simulink model "ScriptDemo"  (R2022b)
settings: configuration reference "TmVcThermal_Configuration_sub" (kept outside this file)
undefined symbols (not defined in the file or in its folder): aaaa, bbbb, cTmComprCtrl_D_u8HvacFlowTable_db, cTmComprCtrl_D_u8HvacFlowTable_sw, cTmComprCtrl_n_i16ChillCmpIMax, cTmComprCtrl_n_i16ChillCmpIMin, cTmComprCtrl_n_i16ChillCmpIMin666, cTmComprCtrl_n_i16ChillCmpPMax, cTmComprCtrl_n_i16ChillCmpPMin, cTmComprCtrl_n_i16CmpChillCoolRpmKiMax, cTmComprCtrl_n_i16CmpChillCoolRpmKiMin, cTmComprCtrl_n_i16CmpChillCoolRpmKpMax, cTmComprCtrl_n_i16CmpChillCoolRpmKpMin, cTmComprCtrl_n_i16CmpCoolRpmKiMax, cTmComprCtrl_n_i16CmpCoolRpmKiMin, cTmComprCtrl_n_i16CmpCoolRpmKpMax, cTmComprCtrl_n_i16CmpCoolRpmKpMin, cTmComprCtrl_n_i16SM4CmpHeatKiMax, cTmComprCtrl_n_i16SM4CmpHeatKiMin, cTmComprCtrl_n_i16SM4CmpHeatKpMax, cTmComprCtrl_n_i16SM4CmpHeatKpMin, cTmComprCtrl_n_i16SM5CmpHeatKiMax, cTmComprCtrl_n_i16SM5CmpHeatKiMin, cTmComprCtrl_n_i16SM5CmpHeatKpMax, cTmComprCtrl_n_i16SM5CmpHeatKpMin, cTmComprCtrl_n_i16SM6CmpHeatKiMax, cTmComprCtrl_n_i16SM6CmpHeatKiMin, cTmComprCtrl_n_i16SM6CmpHeatKpMax, cTmComprCtrl_n_i16SM6CmpHeatKpMin, cTmComprCtrl_n_u16CmpMaxSpdFanFltLimt, cTmComprCtrl_n_u16CmpMaxSpdLoSidePFltLimt, cTmComprCtrl_n_u16CmpMaxSpdSensorFltLimt, cTmComprCtrl_n_u16CompMinRpm, cTmComprCtrl_n_u16CompRpmIncThres, cTmComprCtrl_t_u16BattCooltFFPeriod, cTmComprCtrl_t_u16BattCooltPIPeriod, cTmComprCtrl_t_u16CmpCoolFFPeriod, cTmComprCtrl_t_u16CmpCoolPIPeriod, cTmComprCtrl_t_u16CoolCmpChillFFPeriod, cTmComprCtrl_t_u16CoolCmpChillPIPeriod, cTmComprCtrl_t_u16SM4CmpHeatFFPeriod, cTmComprCtrl_t_u16SM4CmpHeatPIPeriod, cTmComprCtrl_t_u16SM5CmpHeatFFPeriod, cTmComprCtrl_t_u16SM5CmpHeatPIPeriod, cTmComprCtrl_t_u16SM6CmpHeatFFPeriod, cTmComprCtrl_t_u16SM6CmpHeatPIPeriod, cTmComprCtrl_Te_EvapClearInteg, cTmComprCtrl_Te_i16HpReqTempSaturoffset, cTmComprCtrl_Te_i16SatLpReplaceDiff, cTmComprCtrl_Te_i16SM3BatDiffStartEvapDecOffset, cTmComprCtrl_Te_i16SM3EvapLo, cTmComprCtrl_Te_i16SM3TBatDiffEntEvapDecOffset, cTmComprCtrl_Te_i16SM3TBatDiffEntEvapDecOffsetQuit, cTmComprCtrl_Te_s32ErrCmpChillPIContinueCoolH, cTmComprCtrl_Te_s32ErrCmpChillPIContinueCoolL, cTmComprCtrl_Te_s32ErrCmpPIContinueChillH, cTmComprCtrl_Te_s32ErrCmpPIContinueChillL, cTmComprCtrl_Te_s32ErrCmpPIContinueCoolH, cTmComprCtrl_Te_s32ErrCmpPIContinueCoolL, cTmComprCtrl_Te_s32ErrCmpPIContinueHeatH ... (+398)
libraries: simulink x846, PCMULib x711, simulink_need_slupdate x4
(part 19 of 49)

== system ScriptDemo/Create/createBus/createBusGoto/After ==
  note: Before
  note: After
  TmComprCtrl : BusSelector  OutputSignals=Tasks.Task_100ms_TmSw.TmComprCtrl_100,TmDiag_Op.sTmDiag_D_u8BexvFltSt,TmDiag_Op.sTmDiag_D_u8CexvFltSt,TmDiag_Op.sTmDiag_D_u8EexvFltSt,TmDiag_Op.sTmDiag_D_u8FanFltSt,TmDiag_Op.sTmDiag_D_u8HiSidePFltSt,TmDiag_Op.sTmDiag_D_u8LoSidePFltSt,TmDiag_Op.sTmDiag_D_u8OutrCondOutTFltSt,TmDiag_Op.sTmDiag_D_u8Sov1FltSt,TmDiag_Op.sTmDiag_D_u8Sov2FltSt,TmDiag_Op.sTmDiag_D_u8Sov3FltSt,TmDiag_Op.sTmDiag_D_u8Sov4FltSt,TmDiag_Op.sTmDiag_D_u8Sov5FltSt,TmDiag_Op.sTmDiag_D_u8TeEvapFltSt,TmIn_Op.sTmIn_D_u8DCChrgSt,TmIn_Op.sTmIn_D_u8HeatPump,TmIn_Op.sTmIn_D_u8HvActvSts,TmIn_Op.sTmIn_I_s32ElacCmprHvActl,TmIn_Op.sTmIn_Pw_s32HvCoolgAllwd,TmIn_Op.sTmIn_Te_s32BattHv,TmSigProces_Op.sTmSigProces_Te_s32EvapFanReqRamp,TmIn_Op.sTmIn_Te_s32HvBattCooltT,TmIn_Op.sTmIn_Te_s32HvBattCooltTReq,TmIn_Op.sTmIn_U_s32ElacCmprHvActl,TmIn_Op.sTmIn_X_s32BexvPosSts,TmIn_Op.sTmIn_X_s32CexvPosSts,TmIn_Op.sTmIn_X_s32ClimtRcirc,TmIn_Op.sTmIn_X_s32EexvPosSts,TmIn_Op.sTmIn_X_s32HvacTFlpActlPosnFrtRowLe,TmIn_Op.sTmIn_X_s32HvacTFlpActlPosnFrtRowRi,TmIn_Op.sTmIn_n_s32ElacCmprActl,TmIn_Op.sTmIn_v_s32VehSpdLgt,TmRefriModeMgr_Op.sTmRefriModeMgr_D_u8HPCurMode,TmRefriModeMgr_Op.sTmRefriModeMgr_D_u8HpFmCmd,TmRefriModeMgr_Op.sTmRefriModeMgr_D_u8HpModeMainState,TmRefriVlvCtrl_Op.sTmRefriVlvCtrl_Z_u8BEXVInitState,TmRefriVlvCtrl_Op.sTmRefriVlvCtrl_Z_u8CEXVInitState,TmRefriVlvCtrl_Op.sTmRefriVlvCtrl_Z_u8EEXVInitState,TmSigProces_Op.sTmSigProces_D_u8BattThermReq,TmSigProces_Op.sTmSigProces_D_u8HvBattCoolgReq,TmSigProces_Op.sTmSigProces_D_u8PowerFault,TmSigProces_Op.sTmSigProces_Te_s32CompDischarge,TmSigProces_Op.sTmSigProces_Te_s32EvapFanFilter,TmSigProces_Op.sTmSigProces_Te_s32HeatrAirTReqRamp,TmSigProces_Op.sTmSigProces_Te_s32HvBattCooltTFilter,TmSigProces_Op.sTmSigProces_Te_s32HvBattCooltTOutFilter,TmSigProces_Op.sTmSigProces_Te_s32HvacHexAirTFilter,TmSigProces_Op.sTmSigProces_Te_s32TempInlet,TmSigProces_Op.sTmSigProces_Te_s32SatHp,TmSigProces_Op.sTmSigProces_Te_s32SatLp,TmSigProces_Op.sTmSigProces_md_u16BlwHeat,TmSigProces_Op.sTmSigProces_p_u16PHighSide,TmSigProces_Op.sTmSigProces_p_u16PLowSide,TmSovCtrl_Op.sTmSovCtrl_D_u8HpcSov1OnOffSts,TmSovCtrl_Op.sTmSovCtrl_D_u8HpcSov2OnOffSts,TmSovCtrl_Op.sTmSovCtrl_D_u8HpcSov3OnOffSts,TmSovCtrl_Op.sTmSovCtrl_D_u8HpcSov4OnOffSts,TmSovCtrl_Op.sTmSovCtrl_D_u8HpcSov5OnOffSts,TmHvchCtrl_Op.yTmHvchCtrl_B_HpcPtcEnad,TmIn_Op.yTmIn_B_ElAcEnable,TmRefriModeMgr_Op.yTmRefriModeMgr_B_CoolModeInCycle,TmSovCtrl_Op.yTmSovCtrl_B_HpmSov1ActvCmd,TmSovCtrl_Op.yTmSovCtrl_B_HpmSov2ActvCmd,TmSovCtrl_Op.yTmSovCtrl_B_HpmSov3ActvCmd,TmSovCtrl_Op.yTmSovCtrl_B_HpmSov4ActvCmd,TmSovCtrl_Op.yTmSovCtrl_B_HpmSov5ActvCmd,TmDiag_Op.sTmDiag_D_u8AccmFltSt,TmDiag_Op.sTmDiag_D_u8CmprPwrEna2FEnaState,TmDiag_Op.sTmDiag_D_u8CmprSpdEna2FEnaState,TmDiag_Op.sTmDiag_D_u8CmprStsEna2FEnaState,TmDiag_Op.sTmDiag_D_u8CmprStsEnaReq2F,TmDiag_Op.sTmDiag_D_u8HiSidePNHPFltSt,TmDiag_Op.sTmDiag_D_u8HvacHexAirTFltSt,TmDiag_Op.sTmDiag_D_u8InrCondOutTFltSt,TmDiag_Op.sTmDiag_D_u8RefrilackFltSt,TmDiag_Op.sTmDiag_Pw_s32CmprPwrEnaReq2F,TmDiag_Op.sTmDiag_n_s32CmprSpdReq2F,TmDiag_Op.sTmDiag_D_u8CmprDischrgTFltSt,TmSigProces_Op.sTmSigProces_Pw_i16ReqPwrForHeat,TmSigProces_Op.sTmSigProces_md_u16BlwCool,TmSigProces_Op.sTmSigProces_D_u8CarChrgMode,TmIn_Op.sTmIn_D_u8ElecDriveline,TmRefriModeMgr_Op.sTmRefriModeMgr_D_u8CabinCoolReq,TmRefriModeMgr_Op.sTmRefriModeMgr_D_u8CabinHeatReq,TmRefriModeMgr_Op.sTmRefriModeMgr_D_u8HpModeCmd,TmSigProces_Op.sTmSigProces_Te_s32TAmb,TmRefriModeMgr_Op.sTmRefriModeMgr_D_u8ModeSwitchType,TmRefriModeMgr_Op.yTmRefriModeMgr_B_CoolOCRMode,TmDiag_Op.sTmDiag_D_u8BattPmpFltSt,TmDiag_Op.sTmDiag_D_u8HvBattCooltTFltSt,TmDiag_Op.sTmDiag_D_u8HvBattCooltTOutFltSt,TmIn_Op.sTmIn_D_u8OnBdChrgrHndlSts,TmSigProces_Op.sTmSigProces_Pw_i16ReqPwrForCool,TmRefriModeMgr_Op.yTmRefriModeMgr_B_HeatModeInCycle
  TmComprCtrl1 : BusSelector  OutputSignals=Tasks.Task_100ms_TmSw.TmComprCtrl_100,TmDiag_Op.sTmDiag_D_u8BexvFltSt,TmDiag_Op.sTmDiag_D_u8CexvFltSt,TmDiag_Op.sTmDiag_D_u8EexvFltSt,TmDiag_Op.sTmDiag_D_u8FanFltSt,TmDiag_Op.sTmDiag_D_u8HiSidePFltSt,TmDiag_Op.sTmDiag_D_u8LoSidePFltSt,TmDiag_Op.sTmDiag_D_u8OutrCondOutTFltSt,TmDiag_Op.sTmDiag_D_u8Sov1FltSt,TmDiag_Op.sTmDiag_D_u8Sov2FltSt,TmDiag_Op.sTmDiag_D_u8Sov3FltSt,TmDiag_Op.sTmDiag_D_u8Sov4FltSt,TmDiag_Op.sTmDiag_D_u8Sov5FltSt,TmDiag_Op.sTmDiag_D_u8TeEvapFltSt,TmIn_Op.sTmIn_D_u8DCChrgSt,TmIn_Op.sTmIn_D_u8HeatPump,TmIn_Op.sTmIn_D_u8HvActvSts,TmIn_Op.sTmIn_I_s32ElacCmprHvActl,TmIn_Op.sTmIn_Pw_s32HvCoolgAllwd,TmIn_Op.sTmIn_Te_s32BattHv,TmSigProces_Op.sTmSigProces_Te_s32EvapFanReqRamp,TmIn_Op.sTmIn_Te_s32HvBattCooltT,TmIn_Op.sTmIn_Te_s32HvBattCooltTReq,TmIn_Op.sTmIn_U_s32ElacCmprHvActl,TmIn_Op.sTmIn_X_s32BexvPosSts,TmIn_Op.sTmIn_X_s32CexvPosSts,TmIn_Op.sTmIn_X_s32ClimtRcirc,TmIn_Op.sTmIn_X_s32EexvPosSts,TmIn_Op.sTmIn_X_s32HvacTFlpActlPosnFrtRowLe,TmIn_Op.sTmIn_X_s32HvacTFlpActlPosnFrtRowRi,TmIn_Op.sTmIn_n_s32ElacCmprActl,TmIn_Op.sTmIn_v_s32VehSpdLgt,TmRefriModeMgr_Op.sTmRefriModeMgr_D_u8HPCurMode,TmRefriModeMgr_Op.sTmRefriModeMgr_D_u8HpFmCmd,TmRefriModeMgr_Op.sTmRefriModeMgr_D_u8HpModeMainState,TmRefriVlvCtrl_Op.sTmRefriVlvCtrl_Z_u8BEXVInitState,TmRefriVlvCtrl_Op.sTmRefriVlvCtrl_Z_u8CEXVInitState,TmRefriVlvCtrl_Op.sTmRefriVlvCtrl_Z_u8EEXVInitState,TmSigProces_Op.sTmSigProces_D_u8BattThermReq,TmSigProces_Op.sTmSigProces_D_u8HvBattCoolgReq,TmSigProces_Op.sTmSigProces_D_u8PowerFault,TmSigProces_Op.sTmSigProces_Te_s32CompDischarge,TmSigProces_Op.sTmSigProces_Te_s32EvapFanFilter,TmSigProces_Op.sTmSigProces_Te_s32HeatrAirTReqRamp,TmSigProces_Op.sTmSigProces_Te_s32HvBattCooltTFilter,TmSigProces_Op.sTmSigProces_Te_s32HvBattCooltTOutFilter,TmSigProces_Op.sTmSigProces_Te_s32HvacHexAirTFilter,TmSigProces_Op.sTmSigProces_Te_s32TempInlet,TmSigProces_Op.sTmSigProces_Te_s32SatHp,TmSigProces_Op.sTmSigProces_Te_s32SatLp,TmSigProces_Op.sTmSigProces_md_u16BlwHeat,TmSigProces_Op.sTmSigProces_p_u16PHighSide,TmSigProces_Op.sTmSigProces_p_u16PLowSide,TmSovCtrl_Op.sTmSovCtrl_D_u8HpcSov1OnOffSts,TmSovCtrl_Op.sTmSovCtrl_D_u8HpcSov2OnOffSts,TmSovCtrl_Op.sTmSovCtrl_D_u8HpcSov3OnOffSts,TmSovCtrl_Op.sTmSovCtrl_D_u8HpcSov4OnOffSts,TmSovCtrl_Op.sTmSovCtrl_D_u8HpcSov5OnOffSts,TmHvchCtrl_Op.yTmHvchCtrl_B_HpcPtcEnad,TmIn_Op.yTmIn_B_ElAcEnable,TmRefriModeMgr_Op.yTmRefriModeMgr_B_CoolModeInCycle,TmSovCtrl_Op.yTmSovCtrl_B_HpmSov1ActvCmd,TmSovCtrl_Op.yTmSovCtrl_B_HpmSov2ActvCmd,TmSovCtrl_Op.yTmSovCtrl_B_HpmSov3ActvCmd,TmSovCtrl_Op.yTmSovCtrl_B_HpmSov4ActvCmd,TmSovCtrl_Op.yTmSovCtrl_B_HpmSov5ActvCmd,TmDiag_Op.sTmDiag_D_u8AccmFltSt,TmDiag_Op.sTmDiag_D_u8CmprPwrEna2FEnaState,TmDiag_Op.sTmDiag_D_u8CmprSpdEna2FEnaState,TmDiag_Op.sTmDiag_D_u8CmprStsEna2FEnaState,TmDiag_Op.sTmDiag_D_u8CmprStsEnaReq2F,TmDiag_Op.sTmDiag_D_u8HiSidePNHPFltSt,TmDiag_Op.sTmDiag_D_u8HvacHexAirTFltSt,TmDiag_Op.sTmDiag_D_u8InrCondOutTFltSt,TmDiag_Op.sTmDiag_D_u8RefrilackFltSt,TmDiag_Op.sTmDiag_Pw_s32CmprPwrEnaReq2F,TmDiag_Op.sTmDiag_n_s32CmprSpdReq2F,TmDiag_Op.sTmDiag_D_u8CmprDischrgTFltSt,TmSigProces_Op.sTmSigProces_Pw_i16ReqPwrForHeat,TmSigProces_Op.sTmSigProces_md_u16BlwCool,TmSigProces_Op.sTmSigProces_D_u8CarChrgMode,TmIn_Op.sTmIn_D_u8ElecDriveline,TmRefriModeMgr_Op.sTmRefriModeMgr_D_u8CabinCoolReq,TmRefriModeMgr_Op.sTmRefriModeMgr_D_u8CabinHeatReq,TmRefriModeMgr_Op.sTmRefriModeMgr_D_u8HpModeCmd,TmSigProces_Op.sTmSigProces_Te_s32TAmb,TmRefriModeMgr_Op.sTmRefriModeMgr_D_u8ModeSwitchType,TmRefriModeMgr_Op.yTmRefriModeMgr_B_CoolOCRMode,TmDiag_Op.sTmDiag_D_u8BattPmpFltSt,TmDiag_Op.sTmDiag_D_u8HvBattCooltTFltSt,TmDiag_Op.sTmDiag_D_u8HvBattCooltTOutFltSt,TmIn_Op.sTmIn_D_u8OnBdChrgrHndlSts,TmSigProces_Op.sTmSigProces_Pw_i16ReqPwrForCool,TmRefriModeMgr_Op.yTmRefriModeMgr_B_HeatModeInCycle
  wires:
  TmComprCtrl1/1 -> [TmComprCtrl_100]  "<TmComprCtrl_100>"
  TmComprCtrl1/2 -> [sTmDiag_D_u8BexvFltSt]  "<sTmDiag_D_u8BexvFltSt>"
  TmComprCtrl1/3 -> [sTmDiag_D_u8CexvFltSt]  "<sTmDiag_D_u8CexvFltSt>"
  TmComprCtrl1/4 -> [sTmDiag_D_u8EexvFltSt]  "<sTmDiag_D_u8EexvFltSt>"
  TmComprCtrl1/5 -> [sTmDiag_D_u8FanFltSt]  "<sTmDiag_D_u8FanFltSt>"
  TmComprCtrl1/6 -> [sTmDiag_D_u8HiSidePFltSt]  "<sTmDiag_D_u8HiSidePFltSt>"
  TmComprCtrl1/7 -> [sTmDiag_D_u8LoSidePFltSt]  "<sTmDiag_D_u8LoSidePFltSt>"
  TmComprCtrl1/8 -> [sTmDiag_D_u8OutrCondOutTFltSt]  "<sTmDiag_D_u8OutrCondOutTFltSt>"
  TmComprCtrl1/9 -> [sTmDiag_D_u8Sov1FltSt]  "<sTmDiag_D_u8Sov1FltSt>"
  TmComprCtrl1/10 -> [sTmDiag_D_u8Sov2FltSt]  "<sTmDiag_D_u8Sov2FltSt>"
  TmComprCtrl1/11 -> [sTmDiag_D_u8Sov3FltSt]  "<sTmDiag_D_u8Sov3FltSt>"
  TmComprCtrl1/12 -> [sTmDiag_D_u8Sov4FltSt]  "<sTmDiag_D_u8Sov4FltSt>"
  TmComprCtrl1/13 -> [sTmDiag_D_u8Sov5FltSt]  "<sTmDiag_D_u8Sov5FltSt>"
  TmComprCtrl1/14 -> [sTmDiag_D_u8TeEvapFltSt]  "<sTmDiag_D_u8TeEvapFltSt>"
  TmComprCtrl1/15 -> [sTmIn_D_u8DCChrgSt]  "<sTmIn_D_u8DCChrgSt>"
  TmComprCtrl1/16 -> [sTmIn_D_u8HeatPump]  "<sTmIn_D_u8HeatPump>"
  TmComprCtrl1/17 -> [sTmIn_D_u8HvActvSts]  "<sTmIn_D_u8HvActvSts>"
  TmComprCtrl1/18 -> [sTmIn_I_s32ElacCmprHvActl]  "<sTmIn_I_s32ElacCmprHvActl>"
  TmComprCtrl1/19 -> [sTmIn_Pw_s32HvCoolgAllwd]  "<sTmIn_Pw_s32HvCoolgAllwd>"
  TmComprCtrl1/20 -> [sTmIn_Te_s32BattHv]  "<sTmIn_Te_s32BattHv>"
  TmComprCtrl1/21 -> [sTmSigProces_Te_s32EvapFanReqRamp]  "<sTmSigProces_Te_s32EvapFanReqRamp>"
  TmComprCtrl1/22 -> [sTmIn_Te_s32HvBattCooltT]  "<sTmIn_Te_s32HvBattCooltT>"
  TmComprCtrl1/23 -> [sTmIn_Te_s32HvBattCooltTReq]  "<sTmIn_Te_s32HvBattCooltTReq>"
  TmComprCtrl1/24 -> [sTmIn_U_s32ElacCmprHvActl]  "<sTmIn_U_s32ElacCmprHvActl>"
  TmComprCtrl1/25 -> [sTmIn_X_s32BexvPosSts]  "<sTmIn_X_s32BexvPosSts>"
  TmComprCtrl1/26 -> [sTmIn_X_s32CexvPosSts]  "<sTmIn_X_s32CexvPosSts>"
  TmComprCtrl1/27 -> [sTmIn_X_s32ClimtRcirc]  "<sTmIn_X_s32ClimtRcirc>"
  TmComprCtrl1/28 -> [sTmIn_X_s32EexvPosSts]  "<sTmIn_X_s32EexvPosSts>"
  TmComprCtrl1/29 -> [sTmIn_X_s32HvacTFlpActlPosnFrtRowLe]  "<sTmIn_X_s32HvacTFlpActlPosnFrtRowLe>"
  TmComprCtrl1/30 -> [sTmIn_X_s32HvacTFlpActlPosnFrtRowRi]  "<sTmIn_X_s32HvacTFlpActlPosnFrtRowRi>"
  TmComprCtrl1/31 -> [sTmIn_n_s32ElacCmprActl]  "<sTmIn_n_s32ElacCmprActl>"
  TmComprCtrl1/32 -> [sTmIn_v_s32VehSpdLgt]  "<sTmIn_v_s32VehSpdLgt>"
  TmComprCtrl1/33 -> [sTmRefriModeMgr_D_u8HPCurMode]  "<sTmRefriModeMgr_D_u8HPCurMode>"
  TmComprCtrl1/34 -> [sTmRefriModeMgr_D_u8HpFmCmd]  "<sTmRefriModeMgr_D_u8HpFmCmd>"
  TmComprCtrl1/35 -> [sTmRefriModeMgr_D_u8HpModeMainState]  "<sTmRefriModeMgr_D_u8HpModeMainState>"
  TmComprCtrl1/36 -> [sTmRefriVlvCtrl_Z_u8BEXVInitState]  "<sTmRefriVlvCtrl_Z_u8BEXVInitState>"
  TmComprCtrl1/37 -> [sTmRefriVlvCtrl_Z_u8CEXVInitState]  "<sTmRefriVlvCtrl_Z_u8CEXVInitState>"
  TmComprCtrl1/38 -> [sTmRefriVlvCtrl_Z_u8EEXVInitState]  "<sTmRefriVlvCtrl_Z_u8EEXVInitState>"
  TmComprCtrl1/39 -> [sTmSigProces_D_u8BattThermReq]  "<sTmSigProces_D_u8BattThermReq>"
  TmComprCtrl1/40 -> [sTmSigProces_D_u8HvBattCoolgReq]  "<sTmSigProces_D_u8HvBattCoolgReq>"
  TmComprCtrl1/41 -> [sTmSigProces_D_u8PowerFault]  "<sTmSigProces_D_u8PowerFault>"
  TmComprCtrl1/42 -> [sTmSigProces_Te_s32CompDischarge]  "<sTmSigProces_Te_s32CompDischarge>"
  TmComprCtrl1/43 -> [sTmSigProces_Te_s32EvapFanFilter]  "<sTmSigProces_Te_s32EvapFanFilter>"
  TmComprCtrl1/44 -> [sTmSigProces_Te_s32HeatrAirTReqRamp]  "<sTmSigProces_Te_s32HeatrAirTReqRamp>"
  TmComprCtrl1/45 -> [sTmSigProces_Te_s32HvBattCooltTFilter]  "<sTmSigProces_Te_s32HvBattCooltTFilter>"
  TmComprCtrl1/46 -> [sTmSigProces_Te_s32HvBattCooltTOutFilter]  "<sTmSigProces_Te_s32HvBattCooltTOutFilter>"
  TmComprCtrl1/47 -> [sTmSigProces_Te_s32HvacHexAirTFilter]  "<sTmSigProces_Te_s32HvacHexAirTFilter>"
  TmComprCtrl1/48 -> [sTmSigProces_Te_s32TempInlet]  "<sTmSigProces_Te_s32TempInlet>"
  TmComprCtrl1/49 -> [sTmSigProces_Te_s32SatHp]  "<sTmSigProces_Te_s32SatHp>"
  TmComprCtrl1/50 -> [sTmSigProces_Te_s32SatLp]  "<sTmSigProces_Te_s32SatLp>"
  TmComprCtrl1/51 -> [sTmSigProces_md_u16BlwHeat]  "<sTmSigProces_md_u16BlwHeat>"
  TmComprCtrl1/52 -> [sTmSigProces_p_u16PHighSide]  "<sTmSigProces_p_u16PHighSide>"
  TmComprCtrl1/53 -> [sTmSigProces_p_u16PLowSide]  "<sTmSigProces_p_u16PLowSide>"
  TmComprCtrl1/54 -> [sTmSovCtrl_D_u8HpcSov1OnOffSts]  "<sTmSovCtrl_D_u8HpcSov1OnOffSts>"
  TmComprCtrl1/55 -> [sTmSovCtrl_D_u8HpcSov2OnOffSts]  "<sTmSovCtrl_D_u8HpcSov2OnOffSts>"
  TmComprCtrl1/56 -> [sTmSovCtrl_D_u8HpcSov3OnOffSts]  "<sTmSovCtrl_D_u8HpcSov3OnOffSts>"
  TmComprCtrl1/57 -> [sTmSovCtrl_D_u8HpcSov4OnOffSts]  "<sTmSovCtrl_D_u8HpcSov4OnOffSts>"
  TmComprCtrl1/58 -> [sTmSovCtrl_D_u8HpcSov5OnOffSts]  "<sTmSovCtrl_D_u8HpcSov5OnOffSts>"
  TmComprCtrl1/59 -> [yTmHvchCtrl_B_HpcPtcEnad]  "<yTmHvchCtrl_B_HpcPtcEnad>"
  TmComprCtrl1/60 -> [yTmIn_B_ElAcEnable]  "<yTmIn_B_ElAcEnable>"
  TmComprCtrl1/61 -> [yTmRefriModeMgr_B_CoolModeInCycle]  "<yTmRefriModeMgr_B_CoolModeInCycle>"
  TmComprCtrl1/62 -> [yTmSovCtrl_B_HpmSov1ActvCmd]  "<yTmSovCtrl_B_HpmSov1ActvCmd>"
  TmComprCtrl1/63 -> [yTmSovCtrl_B_HpmSov2ActvCmd]  "<yTmSovCtrl_B_HpmSov2ActvCmd>"
  TmComprCtrl1/64 -> [yTmSovCtrl_B_HpmSov3ActvCmd]  "<yTmSovCtrl_B_HpmSov3ActvCmd>"
  TmComprCtrl1/65 -> [yTmSovCtrl_B_HpmSov4ActvCmd]  "<yTmSovCtrl_B_HpmSov4ActvCmd>"
  TmComprCtrl1/66 -> [yTmSovCtrl_B_HpmSov5ActvCmd]  "<yTmSovCtrl_B_HpmSov5ActvCmd>"
  TmComprCtrl1/67 -> [sTmDiag_D_u8AccmFltSt]  "<sTmDiag_D_u8AccmFltSt>"
  TmComprCtrl1/68 -> [sTmDiag_D_u8CmprPwrEna2FEnaState]  "<sTmDiag_D_u8CmprPwrEna2FEnaState>"
  TmComprCtrl1/69 -> [sTmDiag_D_u8CmprSpdEna2FEnaState]  "<sTmDiag_D_u8CmprSpdEna2FEnaState>"
  TmComprCtrl1/70 -> [sTmDiag_D_u8CmprStsEna2FEnaState]  "<sTmDiag_D_u8CmprStsEna2FEnaState>"
  TmComprCtrl1/71 -> [sTmDiag_D_u8CmprStsEnaReq2F]  "<sTmDiag_D_u8CmprStsEnaReq2F>"
  TmComprCtrl1/72 -> [sTmDiag_D_u8HiSidePNHPFltSt]  "<sTmDiag_D_u8HiSidePNHPFltSt>"
  TmComprCtrl1/73 -> [sTmDiag_D_u8HvacHexAirTFltSt]  "<sTmDiag_D_u8HvacHexAirTFltSt>"
  TmComprCtrl1/74 -> [sTmDiag_D_u8InrCondOutTFltSt]  "<sTmDiag_D_u8InrCondOutTFltSt>"
  TmComprCtrl1/75 -> [sTmDiag_D_u8RefrilackFltSt]  "<sTmDiag_D_u8RefrilackFltSt>"
  TmComprCtrl1/76 -> [sTmDiag_Pw_s32CmprPwrEnaReq2F]  "<sTmDiag_Pw_s32CmprPwrEnaReq2F>"
  TmComprCtrl1/77 -> [sTmDiag_n_s32CmprSpdReq2F]  "<sTmDiag_n_s32CmprSpdReq2F>"
  TmComprCtrl1/78 -> [sTmDiag_D_u8CmprDischrgTFltSt]  "<sTmDiag_D_u8CmprDischrgTFltSt>"
  TmComprCtrl1/79 -> [sTmSigProces_Pw_i16ReqPwrForHeat]  "<sTmSigProces_Pw_i16ReqPwrForHeat>"
  TmComprCtrl1/80 -> [sTmSigProces_md_u16BlwCool]  "<sTmSigProces_md_u16BlwCool>"
  TmComprCtrl1/81 -> [sTmSigProces_D_u8CarChrgMode]  "<sTmSigProces_D_u8CarChrgMode>"
  TmComprCtrl1/82 -> [sTmIn_D_u8ElecDriveline]  "<sTmIn_D_u8ElecDriveline>"
  TmComprCtrl1/83 -> [sTmRefriModeMgr_D_u8CabinCoolReq]  "<sTmRefriModeMgr_D_u8CabinCoolReq>"
  TmComprCtrl1/84 -> [sTmRefriModeMgr_D_u8CabinHeatReq]  "<sTmRefriModeMgr_D_u8CabinHeatReq>"
  TmComprCtrl1/85 -> [sTmRefriModeMgr_D_u8HpModeCmd]  "<sTmRefriModeMgr_D_u8HpModeCmd>"
  TmComprCtrl1/86 -> [sTmSigProces_Te_s32TAmb]  "<sTmSigProces_Te_s32TAmb>"
  TmComprCtrl1/87 -> [sTmRefriModeMgr_D_u8ModeSwitchType]  "<sTmRefriModeMgr_D_u8ModeSwitchType>"
  TmComprCtrl1/88 -> [yTmRefriModeMgr_B_CoolOCRMode]  "<yTmRefriModeMgr_B_CoolOCRMode>"
  TmComprCtrl1/89 -> [sTmDiag_D_u8BattPmpFltSt]  "<sTmDiag_D_u8BattPmpFltSt>"
  TmComprCtrl1/90 -> [sTmDiag_D_u8HvBattCooltTFltSt]  "<sTmDiag_D_u8HvBattCooltTFltSt>"
  TmComprCtrl1/91 -> [sTmDiag_D_u8HvBattCooltTOutFltSt]  "<sTmDiag_D_u8HvBattCooltTOutFltSt>"
  TmComprCtrl1/92 -> [sTmIn_D_u8OnBdChrgrHndlSts]  "<sTmIn_D_u8OnBdChrgrHndlSts>"
  TmComprCtrl1/93 -> [sTmSigProces_Pw_i16ReqPwrForCool]  "<sTmSigProces_Pw_i16ReqPwrForCool>"
  TmComprCtrl1/94 -> [yTmRefriModeMgr_B_HeatModeInCycle]  "<yTmRefriModeMgr_B_HeatModeInCycle>"

== system ScriptDemo/Create/createBus/createBusGoto/Before ==
  TmComprCtrl : BusSelector  OutputSignals=Tasks.Task_100ms_TmSw.TmComprCtrl_100,TmDiag_Op.sTmDiag_D_u8BexvFltSt,TmDiag_Op.sTmDiag_D_u8CexvFltSt,TmDiag_Op.sTmDiag_D_u8EexvFltSt,TmDiag_Op.sTmDiag_D_u8FanFltSt,TmDiag_Op.sTmDiag_D_u8HiSidePFltSt,TmDiag_Op.sTmDiag_D_u8LoSidePFltSt,TmDiag_Op.sTmDiag_D_u8OutrCondOutTFltSt,TmDiag_Op.sTmDiag_D_u8Sov1FltSt,TmDiag_Op.sTmDiag_D_u8Sov2FltSt,TmDiag_Op.sTmDiag_D_u8Sov3FltSt,TmDiag_Op.sTmDiag_D_u8Sov4FltSt,TmDiag_Op.sTmDiag_D_u8Sov5FltSt,TmDiag_Op.sTmDiag_D_u8TeEvapFltSt,TmIn_Op.sTmIn_D_u8DCChrgSt,TmIn_Op.sTmIn_D_u8HeatPump,TmIn_Op.sTmIn_D_u8HvActvSts,TmIn_Op.sTmIn_I_s32ElacCmprHvActl,TmIn_Op.sTmIn_Pw_s32HvCoolgAllwd,TmIn_Op.sTmIn_Te_s32BattHv,TmSigProces_Op.sTmSigProces_Te_s32EvapFanReqRamp,TmIn_Op.sTmIn_Te_s32HvBattCooltT,TmIn_Op.sTmIn_Te_s32HvBattCooltTReq,TmIn_Op.sTmIn_U_s32ElacCmprHvActl,TmIn_Op.sTmIn_X_s32BexvPosSts,TmIn_Op.sTmIn_X_s32CexvPosSts,TmIn_Op.sTmIn_X_s32ClimtRcirc,TmIn_Op.sTmIn_X_s32EexvPosSts,TmIn_Op.sTmIn_X_s32HvacTFlpActlPosnFrtRowLe,TmIn_Op.sTmIn_X_s32HvacTFlpActlPosnFrtRowRi,TmIn_Op.sTmIn_n_s32ElacCmprActl,TmIn_Op.sTmIn_v_s32VehSpdLgt,TmRefriModeMgr_Op.sTmRefriModeMgr_D_u8HPCurMode,TmRefriModeMgr_Op.sTmRefriModeMgr_D_u8HpFmCmd,TmRefriModeMgr_Op.sTmRefriModeMgr_D_u8HpModeMainState,TmRefriVlvCtrl_Op.sTmRefriVlvCtrl_Z_u8BEXVInitState,TmRefriVlvCtrl_Op.sTmRefriVlvCtrl_Z_u8CEXVInitState,TmRefriVlvCtrl_Op.sTmRefriVlvCtrl_Z_u8EEXVInitState,TmSigProces_Op.sTmSigProces_D_u8BattThermReq,TmSigProces_Op.sTmSigProces_D_u8HvBattCoolgReq,TmSigProces_Op.sTmSigProces_D_u8PowerFault,TmSigProces_Op.sTmSigProces_Te_s32CompDischarge,TmSigProces_Op.sTmSigProces_Te_s32EvapFanFilter,TmSigProces_Op.sTmSigProces_Te_s32HeatrAirTReqRamp,TmSigProces_Op.sTmSigProces_Te_s32HvBattCooltTFilter,TmSigProces_Op.sTmSigProces_Te_s32HvBattCooltTOutFilter,TmSigProces_Op.sTmSigProces_Te_s32HvacHexAirTFilter,TmSigProces_Op.sTmSigProces_Te_s32TempInlet,TmSigProces_Op.sTmSigProces_Te_s32SatHp,TmSigProces_Op.sTmSigProces_Te_s32SatLp,TmSigProces_Op.sTmSigProces_md_u16BlwHeat,TmSigProces_Op.sTmSigProces_p_u16PHighSide,TmSigProces_Op.sTmSigProces_p_u16PLowSide,TmSovCtrl_Op.sTmSovCtrl_D_u8HpcSov1OnOffSts,TmSovCtrl_Op.sTmSovCtrl_D_u8HpcSov2OnOffSts,TmSovCtrl_Op.sTmSovCtrl_D_u8HpcSov3OnOffSts,TmSovCtrl_Op.sTmSovCtrl_D_u8HpcSov4OnOffSts,TmSovCtrl_Op.sTmSovCtrl_D_u8HpcSov5OnOffSts,TmHvchCtrl_Op.yTmHvchCtrl_B_HpcPtcEnad,TmIn_Op.yTmIn_B_ElAcEnable,TmRefriModeMgr_Op.yTmRefriModeMgr_B_CoolModeInCycle,TmSovCtrl_Op.yTmSovCtrl_B_HpmSov1ActvCmd,TmSovCtrl_Op.yTmSovCtrl_B_HpmSov2ActvCmd,TmSovCtrl_Op.yTmSovCtrl_B_HpmSov3ActvCmd,TmSovCtrl_Op.yTmSovCtrl_B_HpmSov4ActvCmd,TmSovCtrl_Op.yTmSovCtrl_B_HpmSov5ActvCmd,TmDiag_Op.sTmDiag_D_u8AccmFltSt,TmDiag_Op.sTmDiag_D_u8CmprPwrEna2FEnaState,TmDiag_Op.sTmDiag_D_u8CmprSpdEna2FEnaState,TmDiag_Op.sTmDiag_D_u8CmprStsEna2FEnaState,TmDiag_Op.sTmDiag_D_u8CmprStsEnaReq2F,TmDiag_Op.sTmDiag_D_u8HiSidePNHPFltSt,TmDiag_Op.sTmDiag_D_u8HvacHexAirTFltSt,TmDiag_Op.sTmDiag_D_u8InrCondOutTFltSt,TmDiag_Op.sTmDiag_D_u8RefrilackFltSt,TmDiag_Op.sTmDiag_Pw_s32CmprPwrEnaReq2F,TmDiag_Op.sTmDiag_n_s32CmprSpdReq2F,TmDiag_Op.sTmDiag_D_u8CmprDischrgTFltSt,TmSigProces_Op.sTmSigProces_Pw_i16ReqPwrForHeat,TmSigProces_Op.sTmSigProces_md_u16BlwCool,TmSigProces_Op.sTmSigProces_D_u8CarChrgMode,TmIn_Op.sTmIn_D_u8ElecDriveline,TmRefriModeMgr_Op.sTmRefriModeMgr_D_u8CabinCoolReq,TmRefriModeMgr_Op.sTmRefriModeMgr_D_u8CabinHeatReq,TmRefriModeMgr_Op.sTmRefriModeMgr_D_u8HpModeCmd,TmSigProces_Op.sTmSigProces_Te_s32TAmb,TmRefriModeMgr_Op.sTmRefriModeMgr_D_u8ModeSwitchType,TmRefriModeMgr_Op.yTmRefriModeMgr_B_CoolOCRMode,TmDiag_Op.sTmDiag_D_u8BattPmpFltSt,TmDiag_Op.sTmDiag_D_u8HvBattCooltTFltSt,TmDiag_Op.sTmDiag_D_u8HvBattCooltTOutFltSt,TmIn_Op.sTmIn_D_u8OnBdChrgrHndlSts,TmSigProces_Op.sTmSigProces_Pw_i16ReqPwrForCool,TmRefriModeMgr_Op.yTmRefriModeMgr_B_HeatModeInCycle

== system ScriptDemo/Create/createBus/createBusPort/After ==
  note: Before
  note: After
  TmComprCtrl : BusSelector  OutputSignals=TmSigProces_Op.sTmSigProces_Te_s32TempInlet,TmSigProces_Op.sTmSigProces_Te_s32SatHp,TmSigProces_Op.sTmSigProces_Te_s32SatLp,TmSigProces_Op.sTmSigProces_md_u16BlwHeat,TmSigProces_Op.sTmSigProces_p_u16PHighSide,TmSigProces_Op.sTmSigProces_p_u16PLowSide,TmSovCtrl_Op.sTmSovCtrl_D_u8HpcSov1OnOffSts,TmSovCtrl_Op.sTmSovCtrl_D_u8HpcSov2OnOffSts,TmSovCtrl_Op.sTmSovCtrl_D_u8HpcSov3OnOffSts,TmSovCtrl_Op.sTmSovCtrl_D_u8HpcSov4OnOffSts,TmSovCtrl_Op.sTmSovCtrl_D_u8HpcSov5OnOffSts,TmHvchCtrl_Op.yTmHvchCtrl_B_HpcPtcEnad,TmIn_Op.yTmIn_B_ElAcEnable,TmRefriModeMgr_Op.yTmRefriModeMgr_B_CoolModeInCycle,TmSovCtrl_Op.yTmSovCtrl_B_HpmSov1ActvCmd,TmSovCtrl_Op.yTmSovCtrl_B_HpmSov2ActvCmd,TmSovCtrl_Op.yTmSovCtrl_B_HpmSov3ActvCmd,TmSovCtrl_Op.yTmSovCtrl_B_HpmSov4ActvCmd,TmSovCtrl_Op.yTmSovCtrl_B_HpmSov5ActvCmd,TmDiag_Op.sTmDiag_D_u8AccmFltSt,TmDiag_Op.sTmDiag_D_u8CmprPwrEna2FEnaState,TmDiag_Op.sTmDiag_D_u8CmprSpdEna2FEnaState,TmDiag_Op.sTmDiag_D_u8CmprStsEna2FEnaState,TmDiag_Op.sTmDiag_D_u8CmprStsEnaReq2F,TmDiag_Op.sTmDiag_D_u8HiSidePNHPFltSt,TmDiag_Op.sTmDiag_D_u8HvacHexAirTFltSt,TmDiag_Op.sTmDiag_D_u8InrCondOutTFltSt,TmDiag_Op.sTmDiag_D_u8RefrilackFltSt,TmDiag_Op.sTmDiag_Pw_s32CmprPwrEnaReq2F,TmDiag_Op.sTmDiag_n_s32CmprSpdReq2F,TmDiag_Op.sTmDiag_D_u8CmprDischrgTFltSt,TmSigProces_Op.sTmSigProces_Pw_i16ReqPwrForHeat,TmSigProces_Op.sTmSigProces_md_u16BlwCool,TmSigProces_Op.sTmSigProces_D_u8CarChrgMode,TmIn_Op.sTmIn_D_u8ElecDriveline,TmRefriModeMgr_Op.sTmRefriModeMgr_D_u8CabinCoolReq,TmRefriModeMgr_Op.sTmRefriModeMgr_D_u8CabinHeatReq,TmRefriModeMgr_Op.sTmRefriModeMgr_D_u8HpModeCmd,TmSigProces_Op.sTmSigProces_Te_s32TAmb,TmRefriModeMgr_Op.sTmRefriModeMgr_D_u8ModeSwitchType,TmRefriModeMgr_Op.yTmRefriModeMgr_B_CoolOCRMode,TmDiag_Op.sTmDiag_D_u8BattPmpFltSt,TmDiag_Op.sTmDiag_D_u8HvBattCooltTFltSt,TmDiag_Op.sTmDiag_D_u8HvBattCooltTOutFltSt,TmIn_Op.sTmIn_D_u8OnBdChrgrHndlSts,TmSigProces_Op.sTmSigProces_Pw_i16ReqPwrForCool,TmRefriModeMgr_Op.yTmRefriModeMgr_B_HeatModeInCycle
  TmComprCtrl1 : BusSelector  OutputSignals=TmSigProces_Op.sTmSigProces_Te_s32TempInlet,TmSigProces_Op.sTmSigProces_Te_s32SatHp,TmSigProces_Op.sTmSigProces_Te_s32SatLp,TmSigProces_Op.sTmSigProces_md_u16BlwHeat,TmSigProces_Op.sTmSigProces_p_u16PHighSide,TmSigProces_Op.sTmSigProces_p_u16PLowSide,TmSovCtrl_Op.sTmSovCtrl_D_u8HpcSov1OnOffSts,TmSovCtrl_Op.sTmSovCtrl_D_u8HpcSov2OnOffSts,TmSovCtrl_Op.sTmSovCtrl_D_u8HpcSov3OnOffSts,TmSovCtrl_Op.sTmSovCtrl_D_u8HpcSov4OnOffSts,TmSovCtrl_Op.sTmSovCtrl_D_u8HpcSov5OnOffSts,TmHvchCtrl_Op.yTmHvchCtrl_B_HpcPtcEnad,TmIn_Op.yTmIn_B_ElAcEnable,TmRefriModeMgr_Op.yTmRefriModeMgr_B_CoolModeInCycle,TmSovCtrl_Op.yTmSovCtrl_B_HpmSov1ActvCmd,TmSovCtrl_Op.yTmSovCtrl_B_HpmSov2ActvCmd,TmSovCtrl_Op.yTmSovCtrl_B_HpmSov3ActvCmd,TmSovCtrl_Op.yTmSovCtrl_B_HpmSov4ActvCmd,TmSovCtrl_Op.yTmSovCtrl_B_HpmSov5ActvCmd,TmDiag_Op.sTmDiag_D_u8AccmFltSt,TmDiag_Op.sTmDiag_D_u8CmprPwrEna2FEnaState,TmDiag_Op.sTmDiag_D_u8CmprSpdEna2FEnaState,TmDiag_Op.sTmDiag_D_u8CmprStsEna2FEnaState,TmDiag_Op.sTmDiag_D_u8CmprStsEnaReq2F,TmDiag_Op.sTmDiag_D_u8HiSidePNHPFltSt,TmDiag_Op.sTmDiag_D_u8HvacHexAirTFltSt,TmDiag_Op.sTmDiag_D_u8InrCondOutTFltSt,TmDiag_Op.sTmDiag_D_u8RefrilackFltSt,TmDiag_Op.sTmDiag_Pw_s32CmprPwrEnaReq2F,TmDiag_Op.sTmDiag_n_s32CmprSpdReq2F,TmDiag_Op.sTmDiag_D_u8CmprDischrgTFltSt,TmSigProces_Op.sTmSigProces_Pw_i16ReqPwrForHeat,TmSigProces_Op.sTmSigProces_md_u16BlwCool,TmSigProces_Op.sTmSigProces_D_u8CarChrgMode,TmIn_Op.sTmIn_D_u8ElecDriveline,TmRefriModeMgr_Op.sTmRefriModeMgr_D_u8CabinCoolReq,TmRefriModeMgr_Op.sTmRefriModeMgr_D_u8CabinHeatReq,TmRefriModeMgr_Op.sTmRefriModeMgr_D_u8HpModeCmd,TmSigProces_Op.sTmSigProces_Te_s32TAmb,TmRefriModeMgr_Op.sTmRefriModeMgr_D_u8ModeSwitchType,TmRefriModeMgr_Op.yTmRefriModeMgr_B_CoolOCRMode,TmDiag_Op.sTmDiag_D_u8BattPmpFltSt,TmDiag_Op.sTmDiag_D_u8HvBattCooltTFltSt,TmDiag_Op.sTmDiag_D_u8HvBattCooltTOutFltSt,TmIn_Op.sTmIn_D_u8OnBdChrgrHndlSts,TmSigProces_Op.sTmSigProces_Pw_i16ReqPwrForCool,TmRefriModeMgr_Op.yTmRefriModeMgr_B_HeatModeInCycle
  sTmSigProces_Te_s32SatHp : Outport
  sTmSigProces_Te_s32SatLp : Outport  Port=2
  sTmSigProces_md_u16BlwHeat : Outport  Port=3
  sTmSigProces_p_u16PHighSide : Outport  Port=4
  sTmSigProces_p_u16PLowSide : Outport  Port=5
  sTmSovCtrl_D_u8HpcSov1OnOffSts : Outport  Port=6
  sTmSovCtrl_D_u8HpcSov2OnOffSts : Outport  Port=7
  sTmSovCtrl_D_u8HpcSov3OnOffSts : Outport  Port=8
  sTmSovCtrl_D_u8HpcSov4OnOffSts : Outport  Port=9
  sTmSovCtrl_D_u8HpcSov5OnOffSts : Outport  Port=10
  yTmHvchCtrl_B_HpcPtcEnad : Outport  Port=11
  yTmIn_B_ElAcEnable : Outport  Port=12
  yTmSovCtrl_B_HpmSov1ActvCmd : Outport  Port=13
  yTmSovCtrl_B_HpmSov2ActvCmd : Outport  Port=14
  yTmSovCtrl_B_HpmSov3ActvCmd : Outport  Port=15
  yTmSovCtrl_B_HpmSov4ActvCmd : Outport  Port=16
  yTmSovCtrl_B_HpmSov5ActvCmd : Outport  Port=17
  sTmDiag_D_u8AccmFltSt : Outport  Port=18
  sTmDiag_D_u8CmprPwrEna2FEnaState : Outport  Port=19
  sTmDiag_D_u8CmprSpdEna2FEnaState : Outport  Port=20
  sTmDiag_D_u8CmprStsEna2FEnaState : Outport  Port=21
  sTmDiag_D_u8CmprStsEnaReq2F : Outport  Port=22
  sTmDiag_D_u8HiSidePNHPFltSt : Outport  Port=23
  sTmDiag_D_u8HvacHexAirTFltSt : Outport  Port=24
  sTmDiag_D_u8InrCondOutTFltSt : Outport  Port=25
  sTmDiag_D_u8RefrilackFltSt : Outport  Port=26
  sTmDiag_Pw_s32CmprPwrEnaReq2F : Outport  Port=27
  sTmDiag_n_s32CmprSpdReq2F : Outport  Port=28
  sTmDiag_D_u8CmprDischrgTFltSt : Outport  Port=29
  sTmSigProces_Pw_i16ReqPwrForHeat : Outport  Port=30
  sTmSigProces_md_u16BlwCool : Outport  Port=31
  sTmIn_D_u8ElecDriveline : Outport  Port=32
  sTmRefriModeMgr_D_u8CabinCoolReq : Outport  Port=33
  sTmRefriModeMgr_D_u8CabinHeatReq : Outport  Port=34
  sTmRefriModeMgr_D_u8ModeSwitchType : Outport  Port=35
  yTmRefriModeMgr_B_CoolOCRMode : Outport  Port=36
  sTmDiag_D_u8BattPmpFltSt : Outport  Port=37
  sTmDiag_D_u8HvBattCooltTFltSt : Outport  Port=38
  sTmDiag_D_u8HvBattCooltTOutFltSt : Outport  Port=39
  sTmIn_D_u8OnBdChrgrHndlSts : Outport  Port=40
  sTmSigProces_Pw_i16ReqPwrForCool : Outport  Port=41
  yTmRefriModeMgr_B_HeatModeInCycle : Outport  Port=42
  wires:
  TmComprCtrl1/1 -> ?  "<sTmSigProces_Te_s32TempInlet>"
  TmComprCtrl1/2 -> sTmSigProces_Te_s32SatHp/1  "<sTmSigProces_Te_s32SatHp>"
  TmComprCtrl1/3 -> sTmSigProces_Te_s32SatLp/1  "<sTmSigProces_Te_s32SatLp>"
  TmComprCtrl1/4 -> sTmSigProces_md_u16BlwHeat/1  "<sTmSigProces_md_u16BlwHeat>"
  TmComprCtrl1/5 -> sTmSigProces_p_u16PHighSide/1  "<sTmSigProces_p_u16PHighSide>"
  TmComprCtrl1/6 -> sTmSigProces_p_u16PLowSide/1  "<sTmSigProces_p_u16PLowSide>"
  TmComprCtrl1/7 -> sTmSovCtrl_D_u8HpcSov1OnOffSts/1  "<sTmSovCtrl_D_u8HpcSov1OnOffSts>"
  TmComprCtrl1/8 -> sTmSovCtrl_D_u8HpcSov2OnOffSts/1  "<sTmSovCtrl_D_u8HpcSov2OnOffSts>"
  TmComprCtrl1/9 -> sTmSovCtrl_D_u8HpcSov3OnOffSts/1  "<sTmSovCtrl_D_u8HpcSov3OnOffSts>"
  TmComprCtrl1/10 -> sTmSovCtrl_D_u8HpcSov4OnOffSts/1  "<sTmSovCtrl_D_u8HpcSov4OnOffSts>"
  TmComprCtrl1/11 -> sTmSovCtrl_D_u8HpcSov5OnOffSts/1  "<sTmSovCtrl_D_u8HpcSov5OnOffSts>"
  TmComprCtrl1/12 -> yTmHvchCtrl_B_HpcPtcEnad/1  "<yTmHvchCtrl_B_HpcPtcEnad>"
  TmComprCtrl1/13 -> yTmIn_B_ElAcEnable/1  "<yTmIn_B_ElAcEnable>"
  TmComprCtrl1/14 -> ?  "<yTmRefriModeMgr_B_CoolModeInCycle>"
  TmComprCtrl1/15 -> yTmSovCtrl_B_HpmSov1ActvCmd/1  "<yTmSovCtrl_B_HpmSov1ActvCmd>"
  TmComprCtrl1/16 -> yTmSovCtrl_B_HpmSov2ActvCmd/1  "<yTmSovCtrl_B_HpmSov2ActvCmd>"
  TmComprCtrl1/17 -> yTmSovCtrl_B_HpmSov3ActvCmd/1  "<yTmSovCtrl_B_HpmSov3ActvCmd>"
  TmComprCtrl1/18 -> yTmSovCtrl_B_HpmSov4ActvCmd/1  "<yTmSovCtrl_B_HpmSov4ActvCmd>"
  TmComprCtrl1/19 -> yTmSovCtrl_B_HpmSov5ActvCmd/1  "<yTmSovCtrl_B_HpmSov5ActvCmd>"
  TmComprCtrl1/20 -> sTmDiag_D_u8AccmFltSt/1  "<sTmDiag_D_u8AccmFltSt>"
  TmComprCtrl1/21 -> sTmDiag_D_u8CmprPwrEna2FEnaState/1  "<sTmDiag_D_u8CmprPwrEna2FEnaState>"
  TmComprCtrl1/22 -> sTmDiag_D_u8CmprSpdEna2FEnaState/1  "<sTmDiag_D_u8CmprSpdEna2FEnaState>"
  TmComprCtrl1/23 -> sTmDiag_D_u8CmprStsEna2FEnaState/1  "<sTmDiag_D_u8CmprStsEna2FEnaState>"
  TmComprCtrl1/24 -> sTmDiag_D_u8CmprStsEnaReq2F/1  "<sTmDiag_D_u8CmprStsEnaReq2F>"
  TmComprCtrl1/25 -> sTmDiag_D_u8HiSidePNHPFltSt/1  "<sTmDiag_D_u8HiSidePNHPFltSt>"
  TmComprCtrl1/26 -> sTmDiag_D_u8HvacHexAirTFltSt/1  "<sTmDiag_D_u8HvacHexAirTFltSt>"
  TmComprCtrl1/27 -> sTmDiag_D_u8InrCondOutTFltSt/1  "<sTmDiag_D_u8InrCondOutTFltSt>"
  TmComprCtrl1/28 -> sTmDiag_D_u8RefrilackFltSt/1  "<sTmDiag_D_u8RefrilackFltSt>"
  TmComprCtrl1/29 -> sTmDiag_Pw_s32CmprPwrEnaReq2F/1  "<sTmDiag_Pw_s32CmprPwrEnaReq2F>"
  TmComprCtrl1/30 -> sTmDiag_n_s32CmprSpdReq2F/1  "<sTmDiag_n_s32CmprSpdReq2F>"
  TmComprCtrl1/31 -> sTmDiag_D_u8CmprDischrgTFltSt/1  "<sTmDiag_D_u8CmprDischrgTFltSt>"
  TmComprCtrl1/32 -> sTmSigProces_Pw_i16ReqPwrForHeat/1  "<sTmSigProces_Pw_i16ReqPwrForHeat>"
  TmComprCtrl1/33 -> sTmSigProces_md_u16BlwCool/1  "<sTmSigProces_md_u16BlwCool>"
  TmComprCtrl1/34 -> ?  "<sTmSigProces_D_u8CarChrgMode>"
  TmComprCtrl1/35 -> sTmIn_D_u8ElecDriveline/1  "<sTmIn_D_u8ElecDriveline>"
  TmComprCtrl1/36 -> sTmRefriModeMgr_D_u8CabinCoolReq/1  "<sTmRefriModeMgr_D_u8CabinCoolReq>"
  TmComprCtrl1/37 -> sTmRefriModeMgr_D_u8CabinHeatReq/1  "<sTmRefriModeMgr_D_u8CabinHeatReq>"
  TmComprCtrl1/38 -> ?  "<sTmRefriModeMgr_D_u8HpModeCmd>"
  TmComprCtrl1/39 -> ?  "<sTmSigProces_Te_s32TAmb>"
  TmComprCtrl1/40 -> sTmRefriModeMgr_D_u8ModeSwitchType/1  "<sTmRefriModeMgr_D_u8ModeSwitchType>"
  TmComprCtrl1/41 -> yTmRefriModeMgr_B_CoolOCRMode/1  "<yTmRefriModeMgr_B_CoolOCRMode>"
  TmComprCtrl1/42 -> sTmDiag_D_u8BattPmpFltSt/1  "<sTmDiag_D_u8BattPmpFltSt>"
  TmComprCtrl1/43 -> sTmDiag_D_u8HvBattCooltTFltSt/1  "<sTmDiag_D_u8HvBattCooltTFltSt>"
  TmComprCtrl1/44 -> sTmDiag_D_u8HvBattCooltTOutFltSt/1  "<sTmDiag_D_u8HvBattCooltTOutFltSt>"
  TmComprCtrl1/45 -> sTmIn_D_u8OnBdChrgrHndlSts/1  "<sTmIn_D_u8OnBdChrgrHndlSts>"
  TmComprCtrl1/46 -> sTmSigProces_Pw_i16ReqPwrForCool/1  "<sTmSigProces_Pw_i16ReqPwrForCool>"
  TmComprCtrl1/47 -> yTmRefriModeMgr_B_HeatModeInCycle/1  "<yTmRefriModeMgr_B_HeatModeInCycle>"

== system ScriptDemo/Create/createBus/createBusPort/Before ==
  TmComprCtrl : BusSelector  OutputSignals=Tasks.Task_100ms_TmSw.TmComprCtrl_100,TmDiag_Op.sTmDiag_D_u8BexvFltSt,TmDiag_Op.sTmDiag_D_u8CexvFltSt,TmDiag_Op.sTmDiag_D_u8EexvFltSt,TmDiag_Op.sTmDiag_D_u8FanFltSt,TmDiag_Op.sTmDiag_D_u8HiSidePFltSt,TmDiag_Op.sTmDiag_D_u8LoSidePFltSt,TmDiag_Op.sTmDiag_D_u8OutrCondOutTFltSt,TmDiag_Op.sTmDiag_D_u8Sov1FltSt,TmDiag_Op.sTmDiag_D_u8Sov2FltSt,TmDiag_Op.sTmDiag_D_u8Sov3FltSt,TmDiag_Op.sTmDiag_D_u8Sov4FltSt,TmDiag_Op.sTmDiag_D_u8Sov5FltSt,TmDiag_Op.sTmDiag_D_u8TeEvapFltSt,TmIn_Op.sTmIn_D_u8DCChrgSt,TmIn_Op.sTmIn_D_u8HeatPump,TmIn_Op.sTmIn_D_u8HvActvSts,TmIn_Op.sTmIn_I_s32ElacCmprHvActl,TmIn_Op.sTmIn_Pw_s32HvCoolgAllwd,TmIn_Op.sTmIn_Te_s32BattHv,TmSigProces_Op.sTmSigProces_Te_s32EvapFanReqRamp,TmIn_Op.sTmIn_Te_s32HvBattCooltT,TmIn_Op.sTmIn_Te_s32HvBattCooltTReq,TmIn_Op.sTmIn_U_s32ElacCmprHvActl,TmIn_Op.sTmIn_X_s32BexvPosSts,TmIn_Op.sTmIn_X_s32CexvPosSts,TmIn_Op.sTmIn_X_s32ClimtRcirc,TmIn_Op.sTmIn_X_s32EexvPosSts,TmIn_Op.sTmIn_X_s32HvacTFlpActlPosnFrtRowLe,TmIn_Op.sTmIn_X_s32HvacTFlpActlPosnFrtRowRi,TmIn_Op.sTmIn_n_s32ElacCmprActl,TmIn_Op.sTmIn_v_s32VehSpdLgt,TmRefriModeMgr_Op.sTmRefriModeMgr_D_u8HPCurMode,TmRefriModeMgr_Op.sTmRefriModeMgr_D_u8HpFmCmd,TmRefriModeMgr_Op.sTmRefriModeMgr_D_u8HpModeMainState,TmRefriVlvCtrl_Op.sTmRefriVlvCtrl_Z_u8BEXVInitState,TmRefriVlvCtrl_Op.sTmRefriVlvCtrl_Z_u8CEXVInitState,TmRefriVlvCtrl_Op.sTmRefriVlvCtrl_Z_u8EEXVInitState,TmSigProces_Op.sTmSigProces_D_u8BattThermReq,TmSigProces_Op.sTmSigProces_D_u8HvBattCoolgReq,TmSigProces_Op.sTmSigProces_D_u8PowerFault,TmSigProces_Op.sTmSigProces_Te_s32CompDischarge,TmSigProces_Op.sTmSigProces_Te_s32EvapFanFilter,TmSigProces_Op.sTmSigProces_Te_s32HeatrAirTReqRamp,TmSigProces_Op.sTmSigProces_Te_s32HvBattCooltTFilter,TmSigProces_Op.sTmSigProces_Te_s32HvBattCooltTOutFilter,TmSigProces_Op.sTmSigProces_Te_s32HvacHexAirTFilter,TmSigProces_Op.sTmSigProces_Te_s32TempInlet,TmSigProces_Op.sTmSigProces_Te_s32SatHp,TmSigProces_Op.sTmSigProces_Te_s32SatLp,TmSigProces_Op.sTmSigProces_md_u16BlwHeat,TmSigProces_Op.sTmSigProces_p_u16PHighSide,TmSigProces_Op.sTmSigProces_p_u16PLowSide,TmSovCtrl_Op.sTmSovCtrl_D_u8HpcSov1OnOffSts,TmSovCtrl_Op.sTmSovCtrl_D_u8HpcSov2OnOffSts,TmSovCtrl_Op.sTmSovCtrl_D_u8HpcSov3OnOffSts,TmSovCtrl_Op.sTmSovCtrl_D_u8HpcSov4OnOffSts,TmSovCtrl_Op.sTmSovCtrl_D_u8HpcSov5OnOffSts,TmHvchCtrl_Op.yTmHvchCtrl_B_HpcPtcEnad,TmIn_Op.yTmIn_B_ElAcEnable,TmRefriModeMgr_Op.yTmRefriModeMgr_B_CoolModeInCycle,TmSovCtrl_Op.yTmSovCtrl_B_HpmSov1ActvCmd,TmSovCtrl_Op.yTmSovCtrl_B_HpmSov2ActvCmd,TmSovCtrl_Op.yTmSovCtrl_B_HpmSov3ActvCmd,TmSovCtrl_Op.yTmSovCtrl_B_HpmSov4ActvCmd,TmSovCtrl_Op.yTmSovCtrl_B_HpmSov5ActvCmd,TmDiag_Op.sTmDiag_D_u8AccmFltSt,TmDiag_Op.sTmDiag_D_u8CmprPwrEna2FEnaState,TmDiag_Op.sTmDiag_D_u8CmprSpdEna2FEnaState,TmDiag_Op.sTmDiag_D_u8CmprStsEna2FEnaState,TmDiag_Op.sTmDiag_D_u8CmprStsEnaReq2F,TmDiag_Op.sTmDiag_D_u8HiSidePNHPFltSt,TmDiag_Op.sTmDiag_D_u8HvacHexAirTFltSt,TmDiag_Op.sTmDiag_D_u8InrCondOutTFltSt,TmDiag_Op.sTmDiag_D_u8RefrilackFltSt,TmDiag_Op.sTmDiag_Pw_s32CmprPwrEnaReq2F,TmDiag_Op.sTmDiag_n_s32CmprSpdReq2F,TmDiag_Op.sTmDiag_D_u8CmprDischrgTFltSt,TmSigProces_Op.sTmSigProces_Pw_i16ReqPwrForHeat,TmSigProces_Op.sTmSigProces_md_u16BlwCool,TmSigProces_Op.sTmSigProces_D_u8CarChrgMode,TmIn_Op.sTmIn_D_u8ElecDriveline,TmRefriModeMgr_Op.sTmRefriModeMgr_D_u8CabinCoolReq,TmRefriModeMgr_Op.sTmRefriModeMgr_D_u8CabinHeatReq,TmRefriModeMgr_Op.sTmRefriModeMgr_D_u8HpModeCmd,TmSigProces_Op.sTmSigProces_Te_s32TAmb,TmRefriModeMgr_Op.sTmRefriModeMgr_D_u8ModeSwitchType,TmRefriModeMgr_Op.yTmRefriModeMgr_B_CoolOCRMode,TmDiag_Op.sTmDiag_D_u8BattPmpFltSt,TmDiag_Op.sTmDiag_D_u8HvBattCooltTFltSt,TmDiag_Op.sTmDiag_D_u8HvBattCooltTOutFltSt,TmIn_Op.sTmIn_D_u8OnBdChrgrHndlSts,TmSigProces_Op.sTmSigProces_Pw_i16ReqPwrForCool,TmRefriModeMgr_Op.yTmRefriModeMgr_B_HeatModeInCycle

== system ScriptDemo/Create/createDebug/After/After ==
  note: % 目的: 为输出端口创建debug 及对应的输入模块
      | [cnt] = createDebug(gcs)
  sTmRefriVlvCtrl_X_s32CEXVPosReqDbgin : Inport  OutDataTypeStr=single
  sTmRefriVlvCtrl_X_s32EEXVPosReqDbgin : Inport  Port=2  OutDataTypeStr=single
  sTmRefriVlvCtrl_X_s32BEXVPosReqDbgin : Inport  Port=3  OutDataTypeStr=single
  yTmRefriVlvCtrl_B_HpcCexvMovEnableDbgin : Inport  Port=4  OutDataTypeStr=boolean
  sTmRefriVlvCtrl_Z_u8CEXVInitStateDbgin : Inport  Port=5  OutDataTypeStr=uint8
  yTmRefriVlvCtrl_B_CexvCalibReqDbgin : Inport  Port=6  OutDataTypeStr=boolean
  yTmRefriVlvCtrl_B_HpcEexvMovEnableDbgin : Inport  Port=7  OutDataTypeStr=boolean
  sTmRefriVlvCtrl_Z_u8EEXVInitStateDbgin : Inport  Port=8  OutDataTypeStr=uint8
  yTmRefriVlvCtrl_B_EexvCalibReqDbgin : Inport  Port=9  OutDataTypeStr=boolean
  yTmRefriVlvCtrl_B_HpcBexvMovEnableDbgin : Inport  Port=10  OutDataTypeStr=boolean
  sTmRefriVlvCtrl_Z_u8BEXVInitStateDbgin : Inport  Port=11  OutDataTypeStr=uint8
  yTmRefriVlvCtrl_B_BexvCalibReqDbgin : Inport  Port=12  OutDataTypeStr=boolean
  sTmRefriVlvCtrl_X_s32SM3BexvMaxPosDbgin : Inport  Port=13  OutDataTypeStr=single
  yTmRefriVlvCtrl_B_EvapBattTLimBexvEnaDbgin : Inport  Port=14  OutDataTypeStr=boolean
  sTmRefriVlvCtrl_D_u8EexvRefriSwitchStDbgin : Inport  Port=15  OutDataTypeStr=uint8
  sTmRefriVlvCtrl_D_u8CexvRefriSwitchStDbgin : Inport  Port=16  OutDataTypeStr=uint8
  sTmRefriVlvCtrl_D_u8BexvRefriSwitchStDbgin : Inport  Port=17  OutDataTypeStr=uint8
  OutDebug : PCMULib/Interface/OutdebugRvs  SWI=cTmRefriVlvCtrl_X_s32CEXVPosReq_sw  DBI=cTmRefriVlvCtrl_X_s32CEXVPosReq_db
      settings: SourceProductName=PCMULib
  OutDebug1 : PCMULib/Interface/OutdebugRvs  SWI=cTmRefriVlvCtrl_X_s32EEXVPosReq_sw  DBI=cTmRefriVlvCtrl_X_s32EEXVPosReq_db
      settings: SourceProductName=PCMULib
  OutDebug10 : PCMULib/Interface/OutdebugRvs  SWI=cTmRefriVlvCtrl_Z_u8BEXVInitState_sw  DBI=cTmRefriVlvCtrl_Z_u8BEXVInitState_db
      settings: SourceProductName=PCMULib
  OutDebug11 : PCMULib/Interface/OutdebugRvs  SWI=cTmRefriVlvCtrl_B_BexvCalibReq_sw  DBI=cTmRefriVlvCtrl_B_BexvCalibReq_db
      settings: SourceProductName=PCMULib
  OutDebug12 : PCMULib/Interface/OutdebugRvs  SWI=cTmRefriVlvCtrl_X_s32SM3BexvMaxPos_sw  DBI=cTmRefriVlvCtrl_X_s32SM3BexvMaxPos_db
      settings: SourceProductName=PCMULib
  OutDebug13 : PCMULib/Interface/OutdebugRvs  SWI=cTmRefriVlvCtrl_B_EvapBattTLimBexvEna_sw  DBI=cTmRefriVlvCtrl_B_EvapBattTLimBexvEna_db
      settings: SourceProductName=PCMULib
  OutDebug14 : PCMULib/Interface/OutdebugRvs  SWI=cTmRefriVlvCtrl_D_u8EexvRefriSwitchSt_sw  DBI=cTmRefriVlvCtrl_D_u8EexvRefriSwitchSt_db
      settings: SourceProductName=PCMULib
  OutDebug15 : PCMULib/Interface/OutdebugRvs  SWI=cTmRefriVlvCtrl_D_u8CexvRefriSwitchSt_sw  DBI=cTmRefriVlvCtrl_D_u8CexvRefriSwitchSt_db
      settings: SourceProductName=PCMULib
  OutDebug16 : PCMULib/Interface/OutdebugRvs  SWI=cTmRefriVlvCtrl_D_u8BexvRefriSwitchSt_sw  DBI=cTmRefriVlvCtrl_D_u8BexvRefriSwitchSt_db
      settings: SourceProductName=PCMULib
  OutDebug2 : PCMULib/Interface/OutdebugRvs  SWI=cTmRefriVlvCtrl_X_s32BEXVPosReq_sw  DBI=cTmRefriVlvCtrl_X_s32BEXVPosReq_db
      settings: SourceProductName=PCMULib
  OutDebug3 : PCMULib/Interface/OutdebugRvs  SWI=cTmRefriVlvCtrl_B_HpcCexvMovEnable_sw  DBI=cTmRefriVlvCtrl_B_HpcCexvMovEnable_db
      settings: SourceProductName=PCMULib
  OutDebug4 : PCMULib/Interface/OutdebugRvs  SWI=cTmRefriVlvCtrl_Z_u8CEXVInitState_sw  DBI=cTmRefriVlvCtrl_Z_u8CEXVInitState_db
      settings: SourceProductName=PCMULib
  OutDebug5 : PCMULib/Interface/OutdebugRvs  SWI=cTmRefriVlvCtrl_B_CexvCalibReq_sw  DBI=cTmRefriVlvCtrl_B_CexvCalibReq_db
      settings: SourceProductName=PCMULib
  OutDebug6 : PCMULib/Interface/OutdebugRvs  SWI=cTmRefriVlvCtrl_B_HpcEexvMovEnable_sw  DBI=cTmRefriVlvCtrl_B_HpcEexvMovEnable_db
      settings: SourceProductName=PCMULib
  OutDebug7 : PCMULib/Interface/OutdebugRvs  SWI=cTmRefriVlvCtrl_Z_u8EEXVInitState_sw  DBI=cTmRefriVlvCtrl_Z_u8EEXVInitState_db
      settings: SourceProductName=PCMULib
  OutDebug8 : PCMULib/Interface/OutdebugRvs  SWI=cTmRefriVlvCtrl_B_EexvCalibReq_sw  DBI=cTmRefriVlvCtrl_B_EexvCalibReq_db
      settings: SourceProductName=PCMULib
  OutDebug9 : PCMULib/Interface/OutdebugRvs  SWI=cTmRefriVlvCtrl_B_HpcBexvMovEnable_sw  DBI=cTmRefriVlvCtrl_B_HpcBexvMovEnable_db
      settings: SourceProductName=PCMULib
  sTmRefriVlvCtrl_X_s32CEXVPosReq : Outport  OutDataTypeStr=single
  sTmRefriVlvCtrl_X_s32EEXVPosReq : Outport  Port=2  OutDataTypeStr=single
  sTmRefriVlvCtrl_X_s32BEXVPosReq : Outport  Port=3  OutDataTypeStr=single
  yTmRefriVlvCtrl_B_HpcCexvMovEnable : Outport  Port=4  OutDataTypeStr=boolean
  sTmRefriVlvCtrl_Z_u8CEXVInitState : Outport  Port=5  OutDataTypeStr=uint8
  yTmRefriVlvCtrl_B_CexvCalibReq : Outport  Port=6  OutDataTypeStr=boolean
  yTmRefriVlvCtrl_B_HpcEexvMovEnable : Outport  Port=7  OutDataTypeStr=boolean
  sTmRefriVlvCtrl_Z_u8EEXVInitState : Outport  Port=8  OutDataTypeStr=uint8
  yTmRefriVlvCtrl_B_EexvCalibReq : Outport  Port=9  OutDataTypeStr=boolean
  yTmRefriVlvCtrl_B_HpcBexvMovEnable : Outport  Port=10  OutDataTypeStr=boolean
  sTmRefriVlvCtrl_Z_u8BEXVInitState : Outport  Port=11  OutDataTypeStr=uint8
  yTmRefriVlvCtrl_B_BexvCalibReq : Outport  Port=12  OutDataTypeStr=boolean
  sTmRefriVlvCtrl_X_s32SM3BexvMaxPos : Outport  Port=13  OutDataTypeStr=single
  yTmRefriVlvCtrl_B_EvapBattTLimBexvEna : Outport  Port=14  OutDataTypeStr=boolean
  sTmRefriVlvCtrl_D_u8EexvRefriSwitchSt : Outport  Port=15  OutDataTypeStr=uint8
  sTmRefriVlvCtrl_D_u8CexvRefriSwitchSt : Outport  Port=16  OutDataTypeStr=uint8
  sTmRefriVlvCtrl_D_u8BexvRefriSwitchSt : Outport  Port=17  OutDataTypeStr=uint8
  wires:
  sTmRefriVlvCtrl_X_s32CEXVPosReqDbgin/1 -> OutDebug/1
  OutDebug/1 -> sTmRefriVlvCtrl_X_s32CEXVPosReq/1
  sTmRefriVlvCtrl_X_s32EEXVPosReqDbgin/1 -> OutDebug1/1
  OutDebug1/1 -> sTmRefriVlvCtrl_X_s32EEXVPosReq/1
  sTmRefriVlvCtrl_X_s32BEXVPosReqDbgin/1 -> OutDebug2/1
  OutDebug2/1 -> sTmRefriVlvCtrl_X_s32BEXVPosReq/1
  yTmRefriVlvCtrl_B_HpcCexvMovEnableDbgin/1 -> OutDebug3/1
  OutDebug3/1 -> yTmRefriVlvCtrl_B_HpcCexvMovEnable/1
  sTmRefriVlvCtrl_Z_u8CEXVInitStateDbgin/1 -> OutDebug4/1
  OutDebug4/1 -> sTmRefriVlvCtrl_Z_u8CEXVInitState/1
  yTmRefriVlvCtrl_B_CexvCalibReqDbgin/1 -> OutDebug5/1
  OutDebug5/1 -> yTmRefriVlvCtrl_B_CexvCalibReq/1
  yTmRefriVlvCtrl_B_HpcEexvMovEnableDbgin/1 -> OutDebug6/1
  OutDebug6/1 -> yTmRefriVlvCtrl_B_HpcEexvMovEnable/1
  sTmRefriVlvCtrl_Z_u8EEXVInitStateDbgin/1 -> OutDebug7/1
  OutDebug7/1 -> sTmRefriVlvCtrl_Z_u8EEXVInitState/1
  yTmRefriVlvCtrl_B_EexvCalibReqDbgin/1 -> OutDebug8/1
  OutDebug8/1 -> yTmRefriVlvCtrl_B_EexvCalibReq/1
  yTmRefriVlvCtrl_B_HpcBexvMovEnableDbgin/1 -> OutDebug9/1
  OutDebug9/1 -> yTmRefriVlvCtrl_B_HpcBexvMovEnable/1
  sTmRefriVlvCtrl_Z_u8BEXVInitStateDbgin/1 -> OutDebug10/1
  OutDebug10/1 -> sTmRefriVlvCtrl_Z_u8BEXVInitState/1
  yTmRefriVlvCtrl_B_BexvCalibReqDbgin/1 -> OutDebug11/1
  OutDebug11/1 -> yTmRefriVlvCtrl_B_BexvCalibReq/1
  sTmRefriVlvCtrl_X_s32SM3BexvMaxPosDbgin/1 -> OutDebug12/1
  OutDebug12/1 -> sTmRefriVlvCtrl_X_s32SM3BexvMaxPos/1
  yTmRefriVlvCtrl_B_EvapBattTLimBexvEnaDbgin/1 -> OutDebug13/1
  OutDebug13/1 -> yTmRefriVlvCtrl_B_EvapBattTLimBexvEna/1
  sTmRefriVlvCtrl_D_u8EexvRefriSwitchStDbgin/1 -> OutDebug14/1
  OutDebug14/1 -> sTmRefriVlvCtrl_D_u8EexvRefriSwitchSt/1
  sTmRefriVlvCtrl_D_u8CexvRefriSwitchStDbgin/1 -> OutDebug15/1
  OutDebug15/1 -> sTmRefriVlvCtrl_D_u8CexvRefriSwitchSt/1
  sTmRefriVlvCtrl_D_u8BexvRefriSwitchStDbgin/1 -> OutDebug16/1
  OutDebug16/1 -> sTmRefriVlvCtrl_D_u8BexvRefriSwitchSt/1

== system ScriptDemo/Create/createGotoUseless/After/After ==
  sTmDiag_D_u8FanFltSt : Inport  OutDataTypeStr=uint8
  sTmDiag_D_u8HiSidePFltSt : Inport  Port=2  OutDataTypeStr=uint8
  sTmRefriVlvCtrl_Z_u8CEXVInitState : Inport  Port=3  OutDataTypeStr=uint8
  sTmRefriVlvCtrl_Z_u8EEXVInitState : Inport  Port=4  OutDataTypeStr=uint8
  sTmSigProces_D_u8BattThermReq : Inport  Port=5  OutDataTypeStr=uint8
  sTmSigProces_D_u8HvBattCoolgReq : Inport  Port=6  OutDataTypeStr=uint8
  sTmSigProces_D_u8PowerFault : Inport  Port=7  OutDataTypeStr=uint8
  sTmSigProces_Te_s32CompDischarge : Inport  Port=8  OutDataTypeStr=single
  sTmSigProces_Te_s32EvapFanFilter : Inport  Port=9  OutDataTypeStr=single
  Ground{,1..22,33..42} (33 alike) : Ground
  Terminator{19..42} (24 alike) : Terminator
  TmComprCtrl_100 : Outport
  sTmDiag_D_u8CexvFltSt : Outport  Port=2  OutDataTypeStr=uint8
  sTmDiag_D_u8Sov3FltSt : Outport  Port=3  OutDataTypeStr=uint8
  sTmDiag_D_u8Sov5FltSt : Outport  Port=4  OutDataTypeStr=uint8
  sTmDiag_D_u8TeEvapFltSt : Outport  Port=5  OutDataTypeStr=uint8
  sTmIn_D_u8DCChrgSt : Outport  Port=6  OutDataTypeStr=uint8
  sTmIn_D_u8HeatPump : Outport  Port=7  OutDataTypeStr=uint8
  sTmIn_D_u8HvActvSts : Outport  Port=8  OutDataTypeStr=uint8
  sTmIn_I_s32ElacCmprHvActl : Outport  Port=9  OutDataTypeStr=single
  sTmIn_Pw_s32HvCoolgAllwd : Outport  Port=10  OutDataTypeStr=single
  sTmIn_Te_s32BattHv : Outport  Port=11  OutDataTypeStr=single
  sTmIn_Te_s32HvBattCooltT : Outport  Port=12  OutDataTypeStr=single
  sTmIn_U_s32ElacCmprHvActl : Outport  Port=13  OutDataTypeStr=single
  sTmIn_X_s32BexvPosSts : Outport  Port=14  OutDataTypeStr=single
  sTmIn_X_s32CexvPosSts : Outport  Port=15  OutDataTypeStr=single
  sTmSigProces_Te_s32EvapFanReqRamp : Outport  Port=16  OutDataTypeStr=single
  wires:
  [sTmIn_X_s32ClimtRcirc] -> Terminator19/1
  [sTmIn_X_s32EexvPosSts] -> Terminator20/1
  [sTmIn_X_s32HvacTFlpActlPosnFrtRowLe] -> Terminator21/1
  [sTmIn_X_s32HvacTFlpActlPosnFrtRowRi] -> Terminator22/1
  [sTmDiag_D_u8EexvFltSt] -> Terminator23/1
  [sTmIn_n_s32ElacCmprActl] -> Terminator24/1
  [sTmIn_v_s32VehSpdLgt] -> Terminator25/1
  [sTmRefriModeMgr_D_u8HPCurMode] -> Terminator26/1
  [sTmRefriModeMgr_D_u8HpFmCmd] -> Terminator27/1
  [sTmRefriModeMgr_D_u8HpModeMainState] -> Terminator28/1
  [sTmRefriVlvCtrl_Z_u8BEXVInitState] -> Terminator29/1
  [sTmRefriVlvCtrl_Z_u8CEXVInitState] -> Terminator30/1
  [sTmRefriVlvCtrl_Z_u8EEXVInitState] -> Terminator31/1
  [sTmSigProces_D_u8BattThermReq] -> Terminator32/1
  [sTmSigProces_D_u8HvBattCoolgReq] -> Terminator33/1
  [sTmDiag_D_u8FanFltSt] -> Terminator34/1
  [sTmSigProces_D_u8PowerFault] -> Terminator35/1
  [sTmSigProces_Te_s32CompDischarge] -> Terminator36/1
  [sTmSigProces_Te_s32EvapFanFilter] -> Terminator37/1
  [sTmDiag_D_u8HiSidePFltSt] -> Terminator38/1
  [sTmDiag_D_u8LoSidePFltSt] -> Terminator39/1
  [sTmDiag_D_u8OutrCondOutTFltSt] -> Terminator40/1
  [sTmDiag_D_u8Sov1FltSt] -> Terminator41/1
  [sTmDiag_D_u8Sov2FltSt] -> Terminator42/1
  Ground/1 -> [TmComprCtrl_100]
  Ground1/1 -> [sTmDiag_D_u8BexvFltSt]
  Ground2/1 -> [sTmIn_Pw_s32HvCoolgAllwd]
  Ground3/1 -> [sTmIn_Te_s32BattHv]
  Ground4/1 -> [sTmDiag_D_u8CexvFltSt]
  Ground5/1 -> [sTmSigProces_Te_s32EvapFanReqRamp]
  Ground6/1 -> [sTmIn_Te_s32HvBattCooltT]
  Ground7/1 -> [sTmIn_Te_s32HvBattCooltTReq]
  Ground8/1 -> [sTmIn_U_s32ElacCmprHvActl]
  Ground9/1 -> [sTmIn_X_s32BexvPosSts]
  Ground10/1 -> [sTmIn_X_s32CexvPosSts]
  Ground11/1 -> [sTmIn_X_s32ClimtRcirc]
  Ground12/1 -> [sTmDiag_D_u8Sov3FltSt]
  Ground13/1 -> [sTmIn_X_s32EexvPosSts]
  Ground14/1 -> [sTmIn_X_s32HvacTFlpActlPosnFrtRowLe]
  Ground15/1 -> [sTmIn_X_s32HvacTFlpActlPosnFrtRowRi]
  Ground16/1 -> [sTmDiag_D_u8EexvFltSt]
  Ground17/1 -> [sTmIn_n_s32ElacCmprActl]
  Ground18/1 -> [sTmIn_v_s32VehSpdLgt]
  Ground19/1 -> [sTmRefriModeMgr_D_u8HPCurMode]
  Ground20/1 -> [sTmRefriModeMgr_D_u8HpFmCmd]
  Ground21/1 -> [sTmRefriModeMgr_D_u8HpModeMainState]
  Ground22/1 -> [sTmRefriVlvCtrl_Z_u8BEXVInitState]
  Ground33/1 -> [sTmDiag_D_u8LoSidePFltSt]
  Ground34/1 -> [sTmDiag_D_u8Sov5FltSt]
  Ground35/1 -> [sTmDiag_D_u8OutrCondOutTFltSt]
  Ground36/1 -> [sTmDiag_D_u8Sov1FltSt]
  Ground37/1 -> [sTmDiag_D_u8Sov2FltSt]
  Ground38/1 -> [sTmDiag_D_u8TeEvapFltSt]
  Ground39/1 -> [sTmIn_D_u8DCChrgSt]
  Ground40/1 -> [sTmIn_D_u8HeatPump]
  Ground41/1 -> [sTmIn_D_u8HvActvSts]
  Ground42/1 -> [sTmIn_I_s32ElacCmprHvActl]
  sTmDiag_D_u8FanFltSt/1 -> [sTmDiag_D_u8FanFltSt]
  sTmDiag_D_u8HiSidePFltSt/1 -> [sTmDiag_D_u8HiSidePFltSt]
  sTmRefriVlvCtrl_Z_u8CEXVInitState/1 -> [sTmRefriVlvCtrl_Z_u8CEXVInitState]
  sTmRefriVlvCtrl_Z_u8EEXVInitState/1 -> [sTmRefriVlvCtrl_Z_u8EEXVInitState]
  sTmSigProces_D_u8BattThermReq/1 -> [sTmSigProces_D_u8BattThermReq]
  sTmSigProces_D_u8HvBattCoolgReq/1 -> [sTmSigProces_D_u8HvBattCoolgReq]
  sTmSigProces_D_u8PowerFault/1 -> [sTmSigProces_D_u8PowerFault]
  sTmSigProces_Te_s32CompDischarge/1 -> [sTmSigProces_Te_s32CompDischarge]
  sTmSigProces_Te_s32EvapFanFilter/1 -> [sTmSigProces_Te_s32EvapFanFilter]
  [TmComprCtrl_100] -> TmComprCtrl_100/1
  [sTmDiag_D_u8BexvFltSt] -> ?
  [sTmDiag_D_u8CexvFltSt] -> sTmDiag_D_u8CexvFltSt/1
  [sTmDiag_D_u8Sov3FltSt] -> sTmDiag_D_u8Sov3FltSt/1
  [sTmDiag_D_u8Sov5FltSt] -> sTmDiag_D_u8Sov5FltSt/1
  [sTmDiag_D_u8TeEvapFltSt] -> sTmDiag_D_u8TeEvapFltSt/1
  [sTmIn_D_u8DCChrgSt] -> sTmIn_D_u8DCChrgSt/1
  [sTmIn_D_u8HeatPump] -> sTmIn_D_u8HeatPump/1
  [sTmIn_D_u8HvActvSts] -> sTmIn_D_u8HvActvSts/1
  [sTmIn_I_s32ElacCmprHvActl] -> sTmIn_I_s32ElacCmprHvActl/1
  [sTmIn_Pw_s32HvCoolgAllwd] -> sTmIn_Pw_s32HvCoolgAllwd/1
  [sTmIn_Te_s32BattHv] -> sTmIn_Te_s32BattHv/1
  [sTmIn_Te_s32HvBattCooltT] -> sTmIn_Te_s32HvBattCooltT/1
  [sTmIn_Te_s32HvBattCooltTReq] -> ?
  [sTmIn_U_s32ElacCmprHvActl] -> sTmIn_U_s32ElacCmprHvActl/1
  [sTmIn_X_s32BexvPosSts] -> sTmIn_X_s32BexvPosSts/1
  [sTmIn_X_s32CexvPosSts] -> sTmIn_X_s32CexvPosSts/1
  [sTmSigProces_Te_s32EvapFanReqRamp] -> sTmSigProces_Te_s32EvapFanReqRamp/1
